simulink library "DoorRlsReq"  (R2022a)
settings: Solver=VariableStepAuto  StartTime=0.0  StopTime=10.0  RelTol=1e-3
settings Model: Creator=DELL  LastModifiedBy=DELL

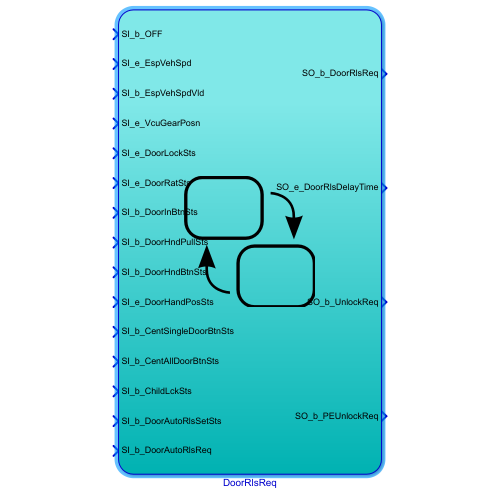
[thumbnail: Simulink's stored preview of the top-level diagram]
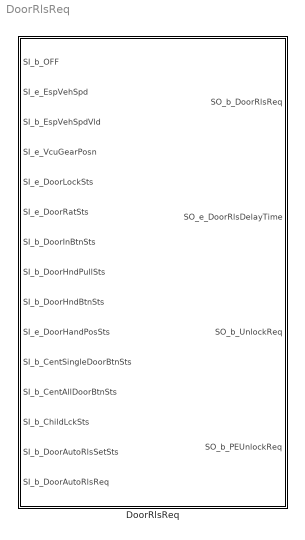
== system DoorRlsReq ==
  DoorRlsReq : Stateflow chart  TreatAsAtomicUnit=on

== stateflow chart DoorRlsReq/DoorRlsReq ==
  state DoorInBtn [parallel]
    settings: executionOrder=1
    state SwValid [parallel]
      settings: executionOrder=1
      state Idle
        en:
        SL_b_DoorInBtnValid = 0;
      state Once
      state Twice
        en:
        SL_b_DoorInBtnValid = 1;
      (default) -> DoorInBtn.SwValid.Idle
      DoorInBtn.SwValid.Idle -> Once : [hasChangedTo(SI_b_DoorInBtnSts, 1)]
      Once -> Twice [order 1] : [hasChangedTo(SI_b_DoorInBtnSts, 1)]
      Once -> DoorInBtn.SwValid.Idle [order 2] : [after(200, tick)]
      Twice -> DoorInBtn.SwValid.Idle : [after(3, tick)]
    state RlsReq [parallel]
      settings: executionOrder=2
      state Idle
        en:
        SL_b_DoorRlsReq1 = 0;
        SO_b_UnlockReq = 0;
      state Trigger
        state DoorLock
          state UnlockReq
            en:
            SO_b_UnlockReq = 1;
            on at(5, tick):
            SO_b_UnlockReq = 0;
          state UnlockSucess
          state UnlockFail
          (default) -> DoorInBtn.RlsReq.Trigger.DoorLock.UnlockReq
          DoorInBtn.RlsReq.Trigger.DoorLock.UnlockReq -> DoorInBtn.RlsReq.Trigger.DoorLock.UnlockFail [order 2] : [after(50, tick) && ...
              | SI_e_DoorLockSts == 0]
          DoorInBtn.RlsReq.Trigger.DoorLock.UnlockReq -> DoorInBtn.RlsReq.Trigger.DoorLock.UnlockSucess [order 1] : [SI_e_DoorLockSts == 1]
        state Release
          en:
          SL_b_DoorRlsReq1 = 1;
          SO_e_DoorRlsDelayTime = 20;
        state DoorUnlock
        state Error
        (default) -> DoorInBtn.RlsReq.Trigger.DoorLock [order 1] : [SI_e_DoorLockSts == 0]
        (default) -> DoorInBtn.RlsReq.Trigger.DoorUnlock [order 2] : [SI_e_DoorLockSts == 1]
        DoorInBtn.RlsReq.Trigger.DoorUnlock -> DoorInBtn.RlsReq.Trigger.Release : [SI_e_DoorRatSts != 3]
        (default) -> DoorInBtn.RlsReq.Trigger.Error [order 3]
        DoorInBtn.RlsReq.Trigger.DoorLock.UnlockSucess -> DoorInBtn.RlsReq.Trigger.Release : [SI_e_DoorRatSts != 3]
      (default) -> DoorInBtn.RlsReq.Idle
      DoorInBtn.RlsReq.Idle -> DoorInBtn.RlsReq.Trigger : [((SI_e_EspVehSpd <= 0 && SI_b_EspVehSpdVld == 0) || ...
          | SI_e_VcuGearPosn == 1) && ...
          | SI_b_ChildLckSts == 0 && ...
          | hasChangedTo(SL_b_DoorInBtnValid, 1)]
      DoorInBtn.RlsReq.Trigger -> DoorInBtn.RlsReq.Idle : [((SI_e_EspVehSpd >= 1 && SI_b_EspVehSpdVld == 0) && ...
          | SI_e_VcuGearPosn != 1) || ...
          | SI_b_ChildLckSts == 1 || ...
          | (SI_e_DoorLockSts == 1 && SI_e_DoorRatSts == 3)]
      DoorInBtn.RlsReq.Trigger.Release -> (junction 173) : [after(5, tick)]
      DoorInBtn.RlsReq.Trigger.Error -> DoorInBtn.RlsReq.Idle
      (junction 173) -> DoorInBtn.RlsReq.Idle
      DoorInBtn.RlsReq.Trigger.DoorLock.UnlockFail -> DoorInBtn.RlsReq.Idle
  state DoorHndPull [parallel]
    settings: executionOrder=2
    state SwValid [parallel]
      settings: executionOrder=1
      state Idle
        en,du:
        SL_b_DoorHndPullValid = SI_b_DoorHndPullSts;
      (default) -> DoorHndPull.SwValid.Idle
    state RlsReq [parallel]
      settings: executionOrder=2
      state Idle
        en:
        SL_b_DoorRlsReq2 = 0;
        SO_b_UnlockReq = 0;
      state Trigger
        state Release
          en:
          SL_b_DoorRlsReq2 = 1;
          SO_e_DoorRlsDelayTime = 4;
        state DoorUnlock
        (default) -> DoorHndPull.RlsReq.Trigger.DoorUnlock
        DoorHndPull.RlsReq.Trigger.DoorUnlock -> DoorHndPull.RlsReq.Trigger.Release : [SI_e_DoorRatSts != 3]
      (default) -> DoorHndPull.RlsReq.Idle
      DoorHndPull.RlsReq.Idle -> DoorHndPull.RlsReq.Trigger : [!SI_b_OFF &&...
          | ((SI_e_EspVehSpd <= 0 && SI_b_EspVehSpdVld == 0) ||...
          | SI_e_VcuGearPosn == 1) &&...
          | SI_e_DoorLockSts == 1 &&...
          | SI_e_DoorHandPosSts == 1 &&...
          | hasChangedTo(SL_b_DoorHndPullValid, 1)]
      DoorHndPull.RlsReq.Trigger -> DoorHndPull.RlsReq.Idle : [SI_b_OFF ||...
          | ((SI_e_EspVehSpd >= 1 && SI_b_EspVehSpdVld == 0) &&...
          | SI_e_VcuGearPosn != 1) ||...
          | SI_e_DoorLockSts != 1 ||...
          | SI_e_DoorHandPosSts != 1 ||...
          | SI_e_DoorRatSts == 3]
      DoorHndPull.RlsReq.Trigger.Release -> (junction 227) : [after(5,tick)]
      (junction 227) -> DoorHndPull.RlsReq.Idle
  state DoorHndBtn [parallel]
    settings: executionOrder=3
    state SwValid [parallel]
      settings: executionOrder=2
      state Idle
        en:
        SL_b_DoorHndBtnValid = 0;
      state Press
      state Release
        en:
        SL_b_DoorHndBtnValid = 1;
      (default) -> DoorHndBtn.SwValid.Idle
      DoorHndBtn.SwValid.Idle -> Press : [hasChangedTo(SI_b_DoorHndBtnSts, 1)]
      Press -> DoorHndBtn.SwValid.Release [order 1] : [hasChangedTo(SI_b_DoorHndBtnSts, 0)]
      Press -> DoorHndBtn.SwValid.Idle [order 2] : [after(100, tick)]
      DoorHndBtn.SwValid.Release -> DoorHndBtn.SwValid.Idle : [after(3, tick)]
    state RlsReq [parallel]
      settings: executionOrder=1
      state Idle
        en:
        SL_b_DoorRlsReq3 = 0;
        SO_b_UnlockReq = 0;
      state Trigger
        state DoorLock
          state UnlockReq
            en:
            SO_b_PEUnlockReq = 1;
            on at(5, tick):
            SO_b_PEUnlockReq = 0;
          state UnlockSucess
          state UnlockFail
          (default) -> DoorHndBtn.RlsReq.Trigger.DoorLock.UnlockReq
          DoorHndBtn.RlsReq.Trigger.DoorLock.UnlockReq -> DoorHndBtn.RlsReq.Trigger.DoorLock.UnlockFail [order 2] : [after(50, tick) && ...
              | SI_e_DoorLockSts == 0]
          DoorHndBtn.RlsReq.Trigger.DoorLock.UnlockReq -> DoorHndBtn.RlsReq.Trigger.DoorLock.UnlockSucess [order 1] : [SI_e_DoorLockSts == 1]
        state Release
          en:
          SL_b_DoorRlsReq3 = 1;
        state DoorUnlock
        state Error
        (default) -> DoorHndBtn.RlsReq.Trigger.DoorLock [order 1] : [SI_e_DoorLockSts == 0]
        (default) -> DoorHndBtn.RlsReq.Trigger.DoorUnlock [order 2] : [SI_e_DoorLockSts == 1]
        DoorHndBtn.RlsReq.Trigger.DoorUnlock -> DoorHndBtn.RlsReq.Trigger.Release : [SI_e_DoorRatSts != 3]
        (default) -> DoorHndBtn.RlsReq.Trigger.Error [order 3]
        DoorHndBtn.RlsReq.Trigger.DoorLock.UnlockSucess -> DoorHndBtn.RlsReq.Trigger.Release : [SI_e_DoorRatSts != 3]
      (default) -> DoorHndBtn.RlsReq.Idle
      DoorHndBtn.RlsReq.Idle -> DoorHndBtn.RlsReq.Trigger : [((SI_e_EspVehSpd <= 0 && SI_b_EspVehSpdVld == 0) ||...
          | SI_e_VcuGearPosn == 1) &&...
          | hasChangedTo(SL_b_DoorHndBtnValid, 1)]
      DoorHndBtn.RlsReq.Trigger -> DoorHndBtn.RlsReq.Idle : [((SI_e_EspVehSpd >= 1 && SI_b_EspVehSpdVld == 0) &&...
          | SI_e_VcuGearPosn != 1) ||...
          | (SI_e_DoorLockSts == 1 && SI_e_DoorRatSts == 3)]
      DoorHndBtn.RlsReq.Trigger.Release -> (junction 265) : [after(5,tick)]
      (junction 265) -> DoorHndBtn.RlsReq.Idle
      DoorHndBtn.RlsReq.Trigger.DoorLock.UnlockFail -> DoorHndBtn.RlsReq.Idle
  state CentDoorBtn [parallel]
    settings: executionOrder=4
    state SwValid [parallel]
      settings: executionOrder=2
      state Idle
        en,du:
        SL_b_CentSingleDoorBtnValid = SI_b_CentSingleDoorBtnSts;
        SL_b_CentAllDoorBtnValid = SI_b_CentAllDoorBtnSts;
      (default) -> CentDoorBtn.SwValid.Idle
    state DoorCentral [parallel]
      settings: executionOrder=1
      state Idle
        en:
        SL_b_DoorRlsReq4 = 0;
        SO_b_UnlockReq = 0;
      state Trigger
        state DoorLock
          state UnlockReq
            en:
            SO_b_UnlockReq = 1;
            on at(5, tick):
            SO_b_UnlockReq = 0;
          state UnlockSucess
          state UnlockFail
          (default) -> CentDoorBtn.DoorCentral.Trigger.DoorLock.UnlockReq
          CentDoorBtn.DoorCentral.Trigger.DoorLock.UnlockReq -> CentDoorBtn.DoorCentral.Trigger.DoorLock.UnlockFail [order 2] : [after(50, tick) && ...
              | SI_e_DoorLockSts == 0]
          CentDoorBtn.DoorCentral.Trigger.DoorLock.UnlockReq -> CentDoorBtn.DoorCentral.Trigger.DoorLock.UnlockSucess [order 1] : [SI_e_DoorLockSts == 1]
        state RELEASE
          en:
          SL_b_DoorRlsReq4 = 1;
        state DoorUnlock
        state Error
        (default) -> CentDoorBtn.DoorCentral.Trigger.DoorLock [order 1] : [SI_e_DoorLockSts == 0]
        (default) -> CentDoorBtn.DoorCentral.Trigger.DoorUnlock [order 2] : [SI_e_DoorLockSts == 1]
        CentDoorBtn.DoorCentral.Trigger.DoorUnlock -> RELEASE : [SI_e_DoorRatSts != 3]
        (default) -> CentDoorBtn.DoorCentral.Trigger.Error [order 3]
        CentDoorBtn.DoorCentral.Trigger.DoorLock.UnlockSucess -> RELEASE : [SI_e_DoorRatSts != 3]
      (default) -> CentDoorBtn.DoorCentral.Idle
      CentDoorBtn.DoorCentral.Idle -> CentDoorBtn.DoorCentral.Trigger : [!SI_b_OFF &&...
          | ((SI_e_EspVehSpd <= 0 && SI_b_EspVehSpdVld == 0) ||...
          | SI_e_VcuGearPosn == 1) &&...
          | (hasChangedTo(SL_b_CentSingleDoorBtnValid, 1) ||...
          | hasChangedTo(SL_b_CentAllDoorBtnValid, 1))]
      CentDoorBtn.DoorCentral.Trigger -> CentDoorBtn.DoorCentral.Idle : [SI_b_OFF ||...
          | ((SI_e_EspVehSpd >= 1 && SI_b_EspVehSpdVld == 0) &&...
          | SI_e_VcuGearPosn != 1) ||...
          | (SI_e_DoorLockSts == 1 && SI_e_DoorRatSts == 3)]
      RELEASE -> (junction 82) : [after(5,tick)]
      CentDoorBtn.DoorCentral.Trigger.Error -> CentDoorBtn.DoorCentral.Idle
      (junction 82) -> CentDoorBtn.DoorCentral.Idle
      CentDoorBtn.DoorCentral.Trigger.DoorLock.UnlockFail -> CentDoorBtn.DoorCentral.Idle
  state DoorAutoRls [parallel]
    settings: executionOrder=5
    state RlsReq [parallel]
      settings: executionOrder=1
      state Idle
        en:
        SL_b_DoorRlsReq5 = 0;
      state Trigger
        state Release
          en:
          SL_b_DoorRlsReq5 = 1;
        state DoorUnlock
        (default) -> DoorAutoRls.RlsReq.Trigger.DoorUnlock
        DoorAutoRls.RlsReq.Trigger.DoorUnlock -> DoorAutoRls.RlsReq.Trigger.Release : [SI_e_DoorRatSts != 3]
      (default) -> DoorAutoRls.RlsReq.Idle
      DoorAutoRls.RlsReq.Idle -> DoorAutoRls.RlsReq.Trigger : [!SI_b_OFF &&...
          | ((SI_e_EspVehSpd <= 0 && SI_b_EspVehSpdVld == 0) || ...
          | SI_e_VcuGearPosn == 1) && ...
          | SI_b_DoorAutoRlsSetSts == 1 && ...
          | SI_e_DoorLockSts == 1 && ...
          | hasChangedTo(SI_b_DoorAutoRlsReq, 1)]
      DoorAutoRls.RlsReq.Trigger -> DoorAutoRls.RlsReq.Idle : [SI_b_OFF ||...
          | ((SI_e_EspVehSpd >= 1 && SI_b_EspVehSpdVld == 0) &&...
          | SI_e_VcuGearPosn != 1) ||...
          | SI_b_DoorAutoRlsSetSts == 0 ||...
          | SI_e_DoorLockSts != 1 ||...
          | SI_e_DoorRatSts == 3]
      DoorAutoRls.RlsReq.Trigger.Release -> (junction 287) : [after(5,tick)]
      (junction 287) -> DoorAutoRls.RlsReq.Idle
  state Rls [parallel]
    settings: executionOrder=6
    (default) -> (junction 487)
    Rls -> (junction 487)
    (junction 487) -> (junction 488) [order 1] : [SL_b_DoorRlsReq1]
    (junction 488) -> (junction 495)
    (junction 487) -> (junction 489) [order 2]
    (junction 489) -> (junction 495) [order 1] : [SL_b_DoorRlsReq2]
    (junction 489) -> (junction 497) [order 2]
    (junction 495) -> (junction 499)
    (junction 497) -> (junction 499) [order 1] : [SL_b_DoorRlsReq3]
    (junction 497) -> (junction 502) [order 2]
    (junction 499) -> (junction 504)
    (junction 502) -> (junction 504) [order 1] : [SL_b_DoorRlsReq4]
    (junction 502) -> (junction 507) [order 2]
    (junction 504) -> (junction 508)
    (junction 507) -> (junction 508) [order 1] : [SL_b_DoorRlsReq5]
    (junction 507) -> (junction 491) [order 2] : {SO_b_DoorRlsReq = 0;}
    (junction 508) -> (junction 493)
    (junction 493) -> (junction 491) : {SO_b_DoorRlsReq = 1;}
    (junction 491) -> (junction 494)
  data: SI_b_OFF input boolean; SI_e_EspVehSpd input uint8; SI_b_EspVehSpdVld input boolean; SI_e_VcuGearPosn input uint8; SO_b_DoorRlsReq output boolean; SO_e_DoorRlsDelayTime output uint8; SI_e_DoorLockSts input uint8; SI_e_DoorRatSts input uint8; SO_b_UnlockReq output boolean; SI_b_DoorInBtnSts input boolean; SI_b_DoorHndPullSts input boolean; SI_b_DoorHndBtnSts input boolean; SI_e_DoorHandPosSts input uint8; SI_b_CentSingleDoorBtnSts input boolean; SI_b_CentAllDoorBtnSts input boolean; SL_b_DoorInBtnValid local boolean; SL_b_CentSingleDoorBtnValid local boolean; SL_b_CentAllDoorBtnValid local boolean; SI_b_ChildLckSts input boolean; SL_b_DoorHndPullValid local boolean; SL_b_DoorHndBtnValid local boolean; SI_b_DoorAutoRlsSetSts input boolean; SI_b_DoorAutoRlsReq input boolean; SO_b_PEUnlockReq output boolean; SL_b_DoorRlsReq1 local boolean; SL_b_DoorRlsReq2 local boolean; SL_b_DoorRlsReq3 local boolean; SL_b_DoorRlsReq4 local boolean; SL_b_DoorRlsReq5 local boolean
